simulink model "slsf_buck"  (R2013a)
settings: Solver=ode45  StartTime=0.0  StopTime=Tmax  RelTol=1e-6
values from neighbouring files (symbols this model uses):
  a00c = -2.339622641509434e+02    (= -233.962264151)    [Buck_Converter.m]
  a00o = -1.962264150943396e+02    (= -196.226415094)    [Buck_Converter.m]
  a01c = -3.773584905660377e+02    (= -377.358490566)    [Buck_Converter.m]
  a01o = -3.773584905660377e+02    (= -377.358490566)    [Buck_Converter.m]
  a10c = 4.545454545454545e+02    (= 454.545454545)    [Buck_Converter.m]
  a10o = 4.545454545454545e+02    (= 454.545454545)    [Buck_Converter.m]
  a11c = -56.818181818181810    (= -56.8181818182)    [Buck_Converter.m]
  a11o = -56.818181818181810    (= -56.8181818182)    [Buck_Converter.m]
  b0c = 1.132075471698113e+04    (= 11320.754717)    [Buck_Converter.m]
  b0o = 0.0    (= 0)    [Buck_Converter.m]
  b1c = 0.0    (= 0)    [Buck_Converter.m]
  b1o = 0.0    (= 0)    [Buck_Converter.m]
  T = 0.00001    (= 1e-05)    [reach_HM.m]
  Vs = 10    [reach_HM.m]
undefined symbols (not defined in the file or in its folder): D, i0, v0, Vs_noise
settings Model: Creator=Omar  LastModifiedBy=omar
settings SolverCC: ZeroCrossControl=EnableAll
settings DataIOCC: SignalLoggingSaveFormat=ModelDataLogs
settings OptimizationCC: ExpressionDepthLimit=2147483647
settings DebuggingCC: MultiTaskDSMMsg=warning  MultiTaskCondExecSysMsg=none
settings RTWCC: IncludeERTFirstTime=on
settings GRTTargetCC: CodeReplacementLibrary=None  CPPClassGenCompliant=on

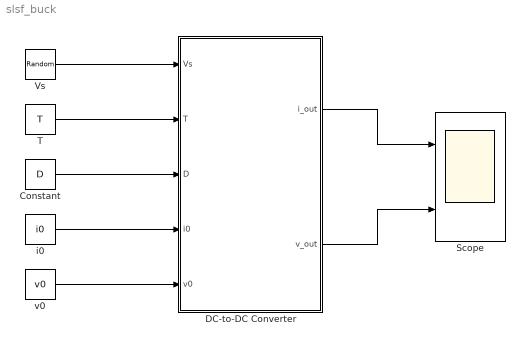
== system slsf_buck ==
  Constant : Constant  Value=D
  DC-to-DC Converter : Stateflow chart  TreatAsAtomicUnit=on
  Scope : Scope  NumInputPorts=2
      settings: YMin=-5~-5  YMax=5~5
  T : Constant  Value=T
  Vs : RandomNumber  Mean=Vs  Variance=Vs_noise  SampleTime=T/10
  i0 : Constant  Value=i0
  v0 : Constant  Value=v0
  wires:
  T/1 -> DC-to-DC Converter/2(T)
  Vs/1 -> DC-to-DC Converter/1(Vs)
  i0/1 -> DC-to-DC Converter/4(i0)
  v0/1 -> DC-to-DC Converter/5(v0)
  Constant/1 -> DC-to-DC Converter/3(D)
  DC-to-DC Converter/1(i_out) -> Scope/1
  DC-to-DC Converter/2(v_out) -> Scope/2

== stateflow chart slsf_buck/DC-to-DC Converter ==
  settings: updateMethod=CONTINUOUS
  state Discontinuous
    du:
    i_dot = a00d*i+a01d*v+b0d*Vs;
    v_dot = a10d*i+a11d*v+b1d*Vs;
    t_dot = 1;
    i_out =i;
    v_out = v;
  state Charging
    du:
    i_dot = a00c*i+a01c*v+b0c*Vs;
    v_dot = a10c*i+a11c*v+b1c*Vs;
    t_dot = 1;
    i_out = i;
    v_out = v;
  state Discharging
    du:
    i_dot = a00o*i+a01o*v+b0o*Vs;
    v_dot = a10o*i+a11o*v+b1o*Vs;
    t_dot = 1;
    i_out = i;
    v_out = v;
  Discharging -> Discontinuous [order 2] : [i<=0]
  Discontinuous -> Charging : [t>= (1-D)*T]
      | {t= 0;}
  Charging -> Discharging : [t>= D*T]
      | {t= 0;}
  Discharging -> Charging [order 1] : [t>= (1-D)*T]
      | {t= 0;}
  (default) -> Charging : {i = i0;
      | v = v0;}
  data: t local double; i local double; a00o local double; Vs input double =120; T input double; D input double; a01o local double; a10o local double; a11o local double; a00c local double; a01c local double; a10c local double; a11c local double; b0o local double; b1o local double; b0c local double; b1c local double; v local double; i0 input double; v0 input double; a01d local double; a10d local double; a11d local double; a00d local double; b0d local double; b1d local double; i_out output double; v_out output double
  data t settings: updateMethod=SF_CONTINUOUS_TIME_DATA
  data i settings: updateMethod=SF_CONTINUOUS_TIME_DATA
  data v settings: updateMethod=SF_CONTINUOUS_TIME_DATA
